simulink model "simulation_model"  (R2023a)
settings: Solver=FixedStepAuto  StartTime=0.0  StopTime=100  FixedStep=ts  RelTol=1e-3
undefined symbols (not defined in the file): a_1, a_2, eta_0, K_p, k_R, k_theta_d, k_theta_p, p, p_0, theta_d
libraries: simulink x2, simulink_extras x1
settings Model: Creator=mori_keigo  LastModifiedBy=mori_keigo

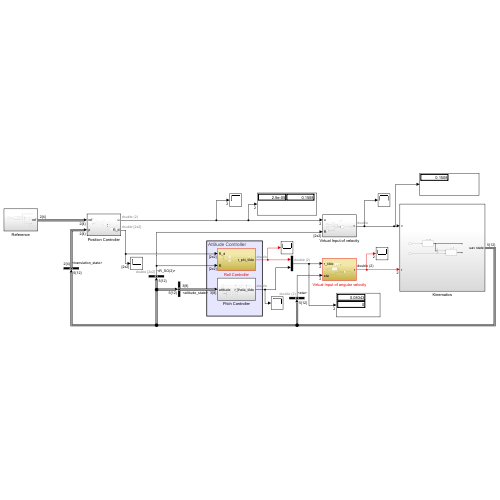
[thumbnail: Simulink's stored preview of the top-level diagram]
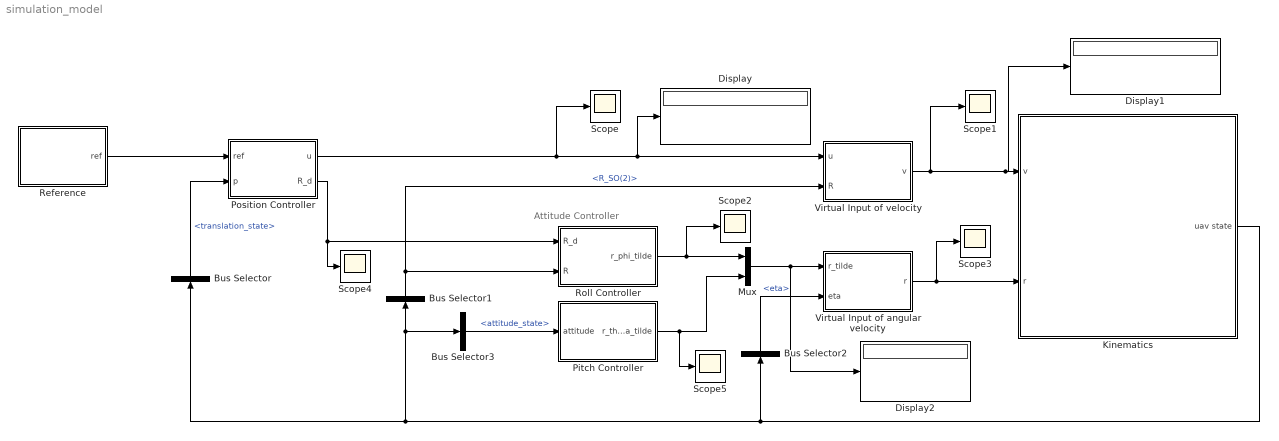
== system simulation_model ==
  note: Attitude Controller
  Bus Selector : BusSelector  OutputSignals=translation_state
  Bus Selector1 : BusSelector  OutputSignals=attitude_state.R_SO(2)
  Bus Selector2 : BusSelector  OutputSignals=attitude_state.eta
  Bus Selector3 : BusSelector  OutputSignals=attitude_state
  Display : Display
  Display1 : Display
  Display2 : Display
  Kinematics : Subsystem
  Mux : Mux  Inputs=2
  Pitch Controller : Subsystem
  Position Controller : Subsystem
  Reference : Subsystem
  Roll Controller : Subsystem
  Scope{,1..5} (6 alike) : Scope
  Virtual Input of angular velocity : Subsystem
  Virtual Input of velocity : Subsystem
  wires:
  Bus Selector/1 -> Position Controller/2(p)  "<translation_state>"
  Reference/1(ref) -> Position Controller/1(ref)
  Position Controller/1(u) -> Scope/1, Display/1, Virtual Input of velocity/1(u)
  Position Controller/2(R_d) -> Scope4/1, Roll Controller/1(R_d)
  Kinematics/1(uav state) -> Bus Selector/1, Bus Selector1/1, Bus Selector3/1, Bus Selector2/1
  Virtual Input of velocity/1(v) -> Display1/1, Kinematics/1(v), Scope1/1
  Roll Controller/1(r_phi_tilde) -> Scope2/1, Mux/1
  Pitch Controller/1(r_theta_tilde) -> Scope5/1, Mux/2
  Mux/1 -> Display2/1, Virtual Input of angular velocity/1(r_tilde)
  Virtual Input of angular velocity/1(r) -> Kinematics/2(r), Scope3/1
  Bus Selector3/1 -> Pitch Controller/1(attitude)  "<attitude_state>"
  Bus Selector1/1 -> Roll Controller/2(R), Virtual Input of velocity/2(R)  "<R_SO(2)>"
  Bus Selector2/1 -> Virtual Input of angular velocity/2(eta)  "<eta>"

== system simulation_model/Kinematics ==
  note: $\dot{\eta} = A \omega$
  note: $\dot{p} = Rv$
  v : Inport
  r : Inport  Port=2
  Bus Selector : BusSelector  OutputSignals=eta
  Kinematics of Attitude : Subsystem
  Kinematics of Translation : Subsystem
  Out Bus Element : Outport  PortName=uav state  Element=attitude_state
  Out Bus Element1 : Outport  PortName=uav state  Element=translation_state
  wires:
  r/1 -> Kinematics of Attitude/1(omega)
  v/1 -> Kinematics of Translation/2(v_z)
  Kinematics of Attitude/1(attitude_state) -> Bus Selector/1, Out Bus Element/1
  Kinematics of Translation/1(uav state) -> Out Bus Element1/1
  Bus Selector/1 -> Kinematics of Translation/1(eta)  "<eta>"

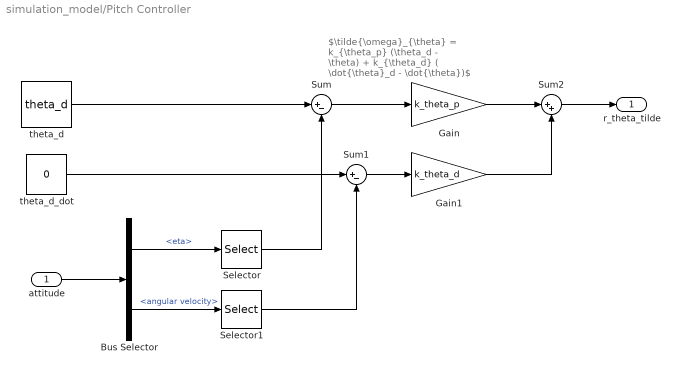
== system simulation_model/Pitch Controller ==
  note: $\tilde{\omega}_{\theta} = k_{\theta_p} (\theta_d - \theta) + k_{\theta_d} ( \dot{\theta}_d - \dot{\theta})$
  attitude : Inport
  Bus Selector : BusSelector  OutputSignals=eta,angular velocity
  Gain : Gain  Gain=k_theta_p
  Gain1 : Gain  Gain=k_theta_d
  Selector : Selector  InputPortWidth=2  IndexOptions=Index vector (dialog)  Indices=[2]  OutputSizes=1
  Selector1 : Selector  InputPortWidth=2  IndexOptions=Index vector (dialog)  Indices=[2]  OutputSizes=1
  Sum : Sum  Inputs=|+-
  Sum1 : Sum  Inputs=|+-
  Sum2 : Sum  Inputs=|++
  theta_d : Constant  Value=theta_d
  theta_d_dot : Constant  Value=0
  r_theta_tilde : Outport
  wires:
  attitude/1 -> Bus Selector/1
  theta_d/1 -> Sum/1
  theta_d_dot/1 -> Sum1/1
  Sum/1 -> Gain/1
  Sum1/1 -> Gain1/1
  Gain/1 -> Sum2/1
  Gain1/1 -> Sum2/2
  Sum2/1 -> r_theta_tilde/1
  Bus Selector/1 -> Selector/1  "<eta>"
  Selector/1 -> Sum/2
  Bus Selector/2 -> Selector1/1  "<angular velocity>"
  Selector1/1 -> Sum1/2

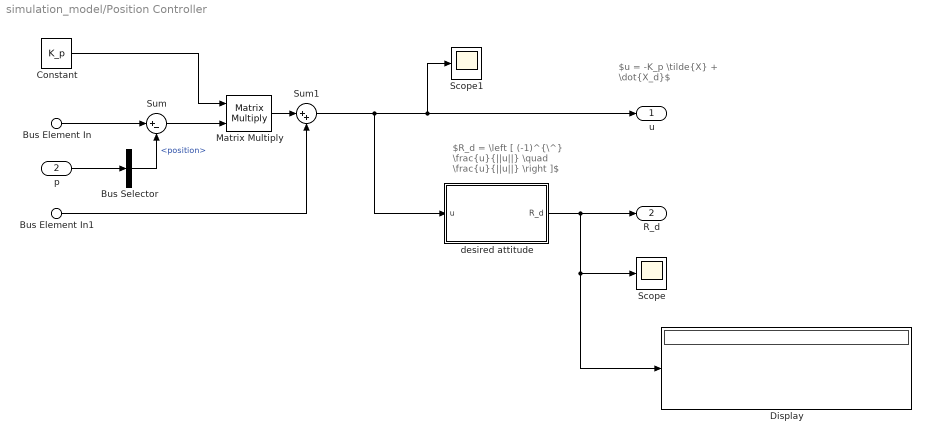
== system simulation_model/Position Controller ==
  note: $u = -K_p \tilde{X} + \dot{X_d}$
  note: $R_d = \left [ (-1)^{\^} \frac{u}{||u||} \quad \frac{u}{||u||} \right ]$
  Bus Element In : Inport  PortName=ref  Element=p_d
  Bus Element In1 : Inport  PortName=ref  Element=p_d_dot
  p : Inport  Port=2
  Bus Selector : BusSelector  OutputSignals=position
  Constant : Constant  Value=K_p
  Display : Display
  Matrix Multiply : Product  Multiplication=Matrix(*)
  Scope : Scope
  Scope1 : Scope
  Sum : Sum  Inputs=|+-
  Sum1 : Sum  Inputs=|++
  desired attitude : Subsystem
  u : Outport
  R_d : Outport  Port=2
  wires:
  Bus Element In/1 -> Sum/1
  Bus Element In1/1 -> Sum1/2
  desired attitude/1(R_d) -> R_d/1, Scope/1, Display/1
  Matrix Multiply/1 -> Sum1/1
  Constant/1 -> Matrix Multiply/1
  Sum/1 -> Matrix Multiply/2
  p/1 -> Bus Selector/1
  Bus Selector/1 -> Sum/2  "<position>"
  Sum1/1 -> u/1, Scope1/1, desired attitude/1(u)

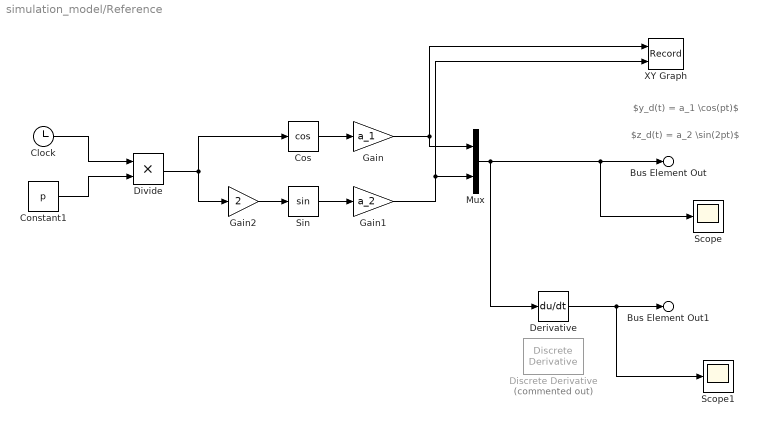
== system simulation_model/Reference ==
  note: $y_d(t) = a_1 \cos(pt)$
  note: $z_d(t) = a_2 \sin(2pt)$
  Clock : Clock
  Constant1 : Constant  Value=p
  Cos : Trigonometry  Operator=cos
  Derivative : Derivative
  Discrete Derivative : simulink/Discrete/Discrete Derivative  Commented=on  gainval=1.0  ICPrevScaledInput=0.0  OutMin=[]  OutMax=[]  OutDataType=fixdt(1, 16)  OutScaling=2^-10  DoSatur=off
  Divide : Product  Inputs=**
  Gain : Gain  Gain=a_1
  Gain1 : Gain  Gain=a_2
  Gain2 : Gain  Gain=2
  Mux : Mux  Inputs=2
  Scope : Scope
  Scope1 : Scope
  Sin : Trigonometry
  XY Graph : Record  FileSettingsInternal="{\"entries\":[{\"content\":{\"excelSettings\":{\"content\":{},\"type\":\"Streamout.ExcelSettings\"}},\"type\":\"Streamout.FileSettingStorage\",\"uuid\":\"\"}],\"packageUris\":[\"http:\\/\\/schema.mathworks.com\\/mf0\\/streamout_blocks\\/R2020a\"],\"version\":\"1.0\"}"  Layout=[1 1]  SignalsInternal="{\"entries\":[{\"content\":{\"signals\":[{\"content\":{\"blockPath\":[],\"dimensions\":[1],\"domain\":\"\",\"lineColor\":\"#a2142f\",\"plots\":[1],\"port\":1,\"sid\":[\"\"],\"signalID\":9636,\"signalName\":\"Gain\"},\"type\":\"RecordBlkView.Signal\",\"uuid\":\"\"},{\"content\":{\"blockPath\":[],\"dimensions\":[1],\"domain\":\"\",\"lineColor\":\"#139fff\",\"plots\":[1],\"port\":2,\"sid\":[\"\"],\"signalID\":9640,\"signalName\":\"Gain1\"},\"type\":\"RecordBlkView.Signal\",\"uuid\":\"\"}]},\"type\":\"RecordBlkView.InputSignals\",\"uuid\":\"\"}],\"packageUris\":[\"http:\\/\\/schema.mathworks.com\\/mf0\\/streamout_blocks\\/R2020a\"],\"version\":\"1.0\"}"  VisualizationBindings="{\"xyplotplugin\":{\"info\":[{\"series\":[{\"bindingParametersList\":[{\"parameter\":\"X-Axis\",\"signalID\":9636,\"signalName\":\"Gain\"},{\"parameter\":\"Y-Axis\",\"signalID\":9640,\"signalName\":\"Gain1\"}],\"seriesID\":31698}],\"subplotID\":1}]}}"  CompatibilityTag=XY
  Bus Element Out : Outport  PortName=ref  Element=p_d
  Bus Element Out1 : Outport  PortName=ref  Element=p_d_dot
  wires:
  Mux/1 -> Derivative/1, Scope/1, Bus Element Out/1
  Cos/1 -> Gain/1
  Sin/1 -> Gain1/1
  Constant1/1 -> Divide/2
  Clock/1 -> Divide/1
  Gain2/1 -> Sin/1
  Divide/1 -> Cos/1, Gain2/1
  Gain1/1 -> Mux/2, XY Graph/2
  Gain/1 -> XY Graph/1, Mux/1
  Derivative/1 -> Scope1/1, Bus Element Out1/1

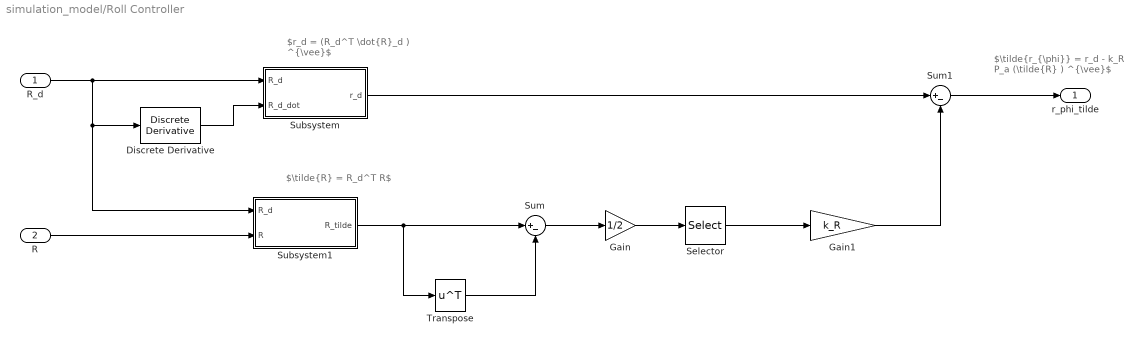
== system simulation_model/Roll Controller ==
  note: $r_d = (R_d^T \dot{R}_d ) ^{\vee}$
  note: $\tilde{r_{\phi}} = r_d - k_R P_a (\tilde{R} ) ^{\vee}$
  note: $\tilde{R} = R_d^T R$
  R_d : Inport
  R : Inport  Port=2
  Discrete Derivative : simulink/Discrete/Discrete Derivative  gainval=1.0  ICPrevScaledInput=0.0  OutMin=[]  OutMax=[]  OutDataType=fixdt(1, 16)  OutScaling=2^-10  DoSatur=off
  Gain : Gain  Gain=1/2
  Gain1 : Gain  Gain=k_R
  Selector : Selector  NumberOfDimensions=2  InputPortWidth=3  IndexOptions=Index vector (dialog),Index vector (dialog)  Indices=[2],1  OutputSizes=1,1
  Subsystem : Subsystem
  Subsystem1 : Subsystem
  Sum : Sum  Inputs=|+-
  Sum1 : Sum  Inputs=|+-
  Transpose : Math  Operator=transpose
  r_phi_tilde : Outport
  wires:
  R_d/1 -> Subsystem1/1(R_d), Discrete Derivative/1, Subsystem/1(R_d)
  Discrete Derivative/1 -> Subsystem/2(R_d_dot)
  R/1 -> Subsystem1/2(R)
  Subsystem1/1(R_tilde) -> Transpose/1, Sum/1
  Transpose/1 -> Sum/2
  Sum/1 -> Gain/1
  Gain/1 -> Selector/1
  Selector/1 -> Gain1/1
  Sum1/1 -> r_phi_tilde/1
  Subsystem/1(r_d) -> Sum1/1
  Gain1/1 -> Sum1/2

== system simulation_model/Virtual Input of angular velocity ==
  note: $r = A^{-1} \tilde{r}$
  r_tilde : Inport
  eta : Inport  Port=2
  Product : Product  Inputs=/*  Multiplication=Matrix(*)
  Transformation to A : Subsystem
  r : Outport
  wires:
  Transformation to A/1(A) -> Product/1
  r_tilde/1 -> Product/2
  Product/1 -> r/1
  eta/1 -> Transformation to A/1(eta)

== system simulation_model/Virtual Input of velocity ==
  note: $v_z = u^T Re_2$
  u : Inport
  R : Inport  Port=2
  Constant : Constant  Value=[0;1]  VectorParams1D=off
  Matrix Multiply : Product  Inputs=3  Multiplication=Matrix(*)
  Transpose : Math  Operator=transpose
  v : Outport
  wires:
  R/1 -> Matrix Multiply/2
  Transpose/1 -> Matrix Multiply/1
  Matrix Multiply/1 -> v/1
  u/1 -> Transpose/1
  Constant/1 -> Matrix Multiply/3

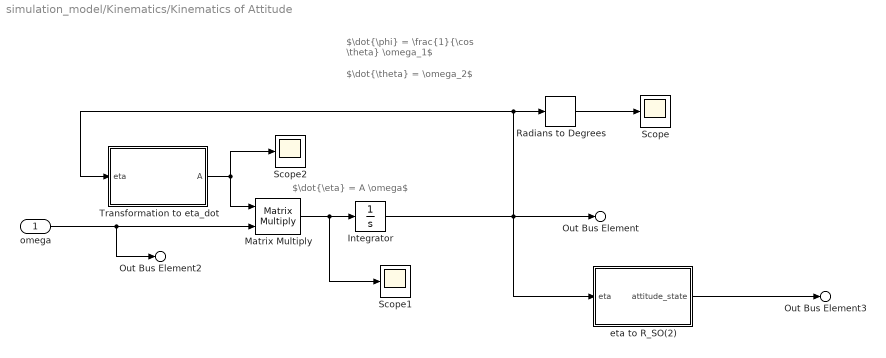
== system simulation_model/Kinematics/Kinematics of Attitude ==
  note: $\dot{\theta} = \omega_2$
  note: $\dot{\phi} = \frac{1}{\cos \theta} \omega_1$
  note: $\dot{\eta} = A \omega$
  omega : Inport
  Integrator : Integrator  InitialCondition=eta_0
  Matrix Multiply : Product  Multiplication=Matrix(*)
  Radians to Degrees : simulink_extras/Transformations/Radians to Degrees
  Scope : Scope
  Scope1 : Scope
  Scope2 : Scope
  Transformation to eta_dot : Subsystem
  eta to R_SO(2) : Subsystem
  Out Bus Element : Outport  PortName=attitude_state  Element=eta
  Out Bus Element2 : Outport  PortName=attitude_state  Element=angular velocity
  Out Bus Element3 : Outport  PortName=attitude_state  Element=R_SO(2)
  wires:
  Integrator/1 -> Out Bus Element/1, eta to R_SO(2)/1(eta), Transformation to eta_dot/1(eta), Radians to Degrees/1
  Matrix Multiply/1 -> Scope1/1, Integrator/1
  omega/1 -> Out Bus Element2/1, Matrix Multiply/2
  Transformation to eta_dot/1(A) -> Matrix Multiply/1, Scope2/1
  Radians to Degrees/1 -> Scope/1
  eta to R_SO(2)/1(attitude_state) -> Out Bus Element3/1

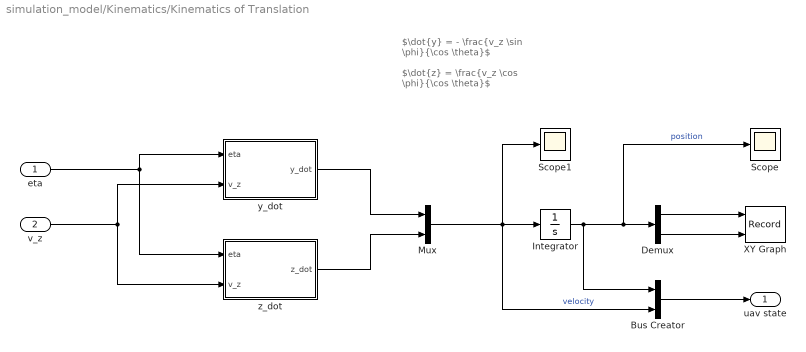
== system simulation_model/Kinematics/Kinematics of Translation ==
  note: $\dot{z} = \frac{v_z \cos \phi}{\cos \theta}$
  note: $\dot{y} = - \frac{v_z \sin \phi}{\cos \theta}$
  eta : Inport
  v_z : Inport  Port=2
  Bus Creator : BusCreator  Inputs=2
  Demux : Demux  Outputs=2
  Integrator : Integrator  InitialCondition=p_0
  Mux : Mux  Inputs=2
  Scope : Scope
  Scope1 : Scope
  XY Graph : Record  FileSettingsInternal="{\"entries\":[{\"content\":{\"excelSettings\":{\"content\":{},\"type\":\"Streamout.ExcelSettings\"}},\"type\":\"Streamout.FileSettingStorage\",\"uuid\":\"\"}],\"packageUris\":[\"http:\\/\\/schema.mathworks.com\\/mf0\\/streamout_blocks\\/R2020a\"],\"version\":\"1.0\"}"  Layout=[1 1]  SignalsInternal="{\"entries\":[{\"content\":{\"signals\":[{\"content\":{\"blockPath\":[],\"dimensions\":[1],\"domain\":\"\",\"lineColor\":\"#a2142f\",\"plots\":[1],\"port\":1,\"sid\":[\"\"],\"signalID\":9628,\"signalName\":\"Demux:1\"},\"type\":\"RecordBlkView.Signal\",\"uuid\":\"\"},{\"content\":{\"blockPath\":[],\"dimensions\":[1],\"domain\":\"\",\"lineColor\":\"#139fff\",\"plots\":[1],\"port\":2,\"sid\":[\"\"],\"signalID\":9632,\"signalName\":\"Demux:2\"},\"type\":\"RecordBlkView.Signal\",\"uuid\":\"\"}]},\"type\":\"RecordBlkView.InputSignals\",\"uuid\":\"\"}],\"packageUris\":[\"http:\\/\\/schema.mathworks.com\\/mf0\\/streamout_blocks\\/R2020a\"],\"version\":\"1.0\"}"  VisualizationBindings="{\"xyplotplugin\":{\"info\":[{\"series\":[{\"bindingParametersList\":[{\"parameter\":\"X-Axis\",\"signalID\":9628,\"signalName\":\"Demux:1\"},{\"parameter\":\"Y-Axis\",\"signalID\":9632,\"signalName\":\"Demux:2\"}],\"seriesID\":17287}],\"subplotID\":1}]}}"  CompatibilityTag=XY
  y_dot : Subsystem
  z_dot : Subsystem
  uav state : Outport
  wires:
  Integrator/1 -> Scope/1, Demux/1, Bus Creator/1  "position"
  Mux/1 -> Scope1/1, Bus Creator/2, Integrator/1  "velocity"
  Bus Creator/1 -> uav state/1
  eta/1 -> z_dot/1(eta), y_dot/1(eta)
  y_dot/1(y_dot) -> Mux/1
  v_z/1 -> z_dot/2(v_z), y_dot/2(v_z)
  z_dot/1(z_dot) -> Mux/2
  Demux/1 -> XY Graph/1
  Demux/2 -> XY Graph/2

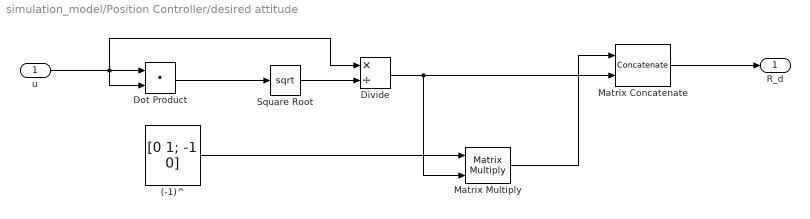
== system simulation_model/Position Controller/desired attitude ==
  u : Inport
  (-1)^ : Constant  Value=[0 1; -1 0]  VectorParams1D=off
  Divide : Product  Inputs=*/
  Dot Product : DotProduct  OutDataTypeStr=Inherit: Inherit via internal rule
  Matrix Concatenate : Concatenate  Mode=Multidimensional array  ConcatenateDimension=2
  Matrix Multiply : Product  Multiplication=Matrix(*)
  Square Root : Sqrt
  R_d : Outport
  wires:
  Dot Product/1 -> Square Root/1
  u/1 -> Divide/1, Dot Product/2, Dot Product/1
  Square Root/1 -> Divide/2
  Matrix Concatenate/1 -> R_d/1
  Divide/1 -> Matrix Concatenate/2, Matrix Multiply/2
  (-1)^/1 -> Matrix Multiply/1
  Matrix Multiply/1 -> Matrix Concatenate/1

== system simulation_model/Roll Controller/Subsystem ==
  R_d : Inport
  R_d_dot : Inport  Port=2
  Matrix Multiply : Product  Multiplication=Matrix(*)
  Selector : Selector  NumberOfDimensions=2  InputPortWidth=3  IndexOptions=Index vector (dialog),Index vector (dialog)  Indices=[2],1  OutputSizes=1,1
  Transpose : Math  Operator=transpose
  r_d : Outport
  wires:
  R_d/1 -> Transpose/1
  Transpose/1 -> Matrix Multiply/1
  R_d_dot/1 -> Matrix Multiply/2
  Matrix Multiply/1 -> Selector/1
  Selector/1 -> r_d/1

== system simulation_model/Roll Controller/Subsystem1 ==
  R_d : Inport
  R : Inport  Port=2
  Matrix Multiply : Product  Multiplication=Matrix(*)
  Transpose : Math  Operator=transpose
  R_tilde : Outport
  wires:
  R_d/1 -> Transpose/1
  Transpose/1 -> Matrix Multiply/1
  R/1 -> Matrix Multiply/2
  Matrix Multiply/1 -> R_tilde/1

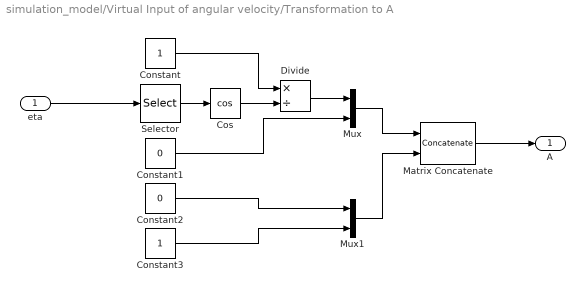
== system simulation_model/Virtual Input of angular velocity/Transformation to A ==
  eta : Inport
  Constant : Constant
  Constant1 : Constant  Value=0
  Constant2 : Constant  Value=0
  Constant3 : Constant
  Cos : Trigonometry  Operator=cos
  Divide : Product  Inputs=*/
  Matrix Concatenate : Concatenate  Mode=Multidimensional array  ConcatenateDimension=2
  Mux : Mux  Inputs=2
  Mux1 : Mux  Inputs=2
  Selector : Selector  InputPortWidth=2  IndexOptions=Index vector (dialog)  Indices=[2]  OutputSizes=1
  A : Outport
  wires:
  eta/1 -> Selector/1
  Constant/1 -> Divide/1
  Divide/1 -> Mux/1
  Constant1/1 -> Mux/2
  Constant2/1 -> Mux1/1
  Constant3/1 -> Mux1/2
  Mux/1 -> Matrix Concatenate/1
  Mux1/1 -> Matrix Concatenate/2
  Matrix Concatenate/1 -> A/1
  Selector/1 -> Cos/1
  Cos/1 -> Divide/2

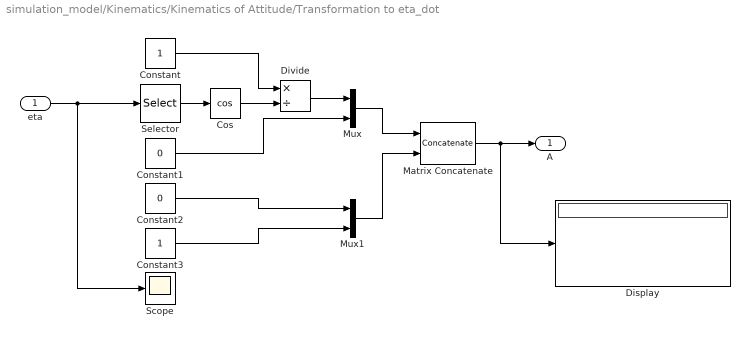
== system simulation_model/Kinematics/Kinematics of Attitude/Transformation to eta_dot ==
  eta : Inport
  Constant : Constant
  Constant1 : Constant  Value=0
  Constant2 : Constant  Value=0
  Constant3 : Constant
  Cos : Trigonometry  Operator=cos
  Display : Display
  Divide : Product  Inputs=*/
  Matrix Concatenate : Concatenate  Mode=Multidimensional array  ConcatenateDimension=2
  Mux : Mux  Inputs=2
  Mux1 : Mux  Inputs=2
  Scope : Scope
  Selector : Selector  InputPortWidth=2  IndexOptions=Index vector (dialog)  Indices=[2]  OutputSizes=1
  A : Outport
  wires:
  eta/1 -> Scope/1, Selector/1
  Constant/1 -> Divide/1
  Divide/1 -> Mux/1
  Constant1/1 -> Mux/2
  Constant2/1 -> Mux1/1
  Constant3/1 -> Mux1/2
  Mux/1 -> Matrix Concatenate/1
  Mux1/1 -> Matrix Concatenate/2
  Matrix Concatenate/1 -> Display/1, A/1
  Selector/1 -> Cos/1
  Cos/1 -> Divide/2

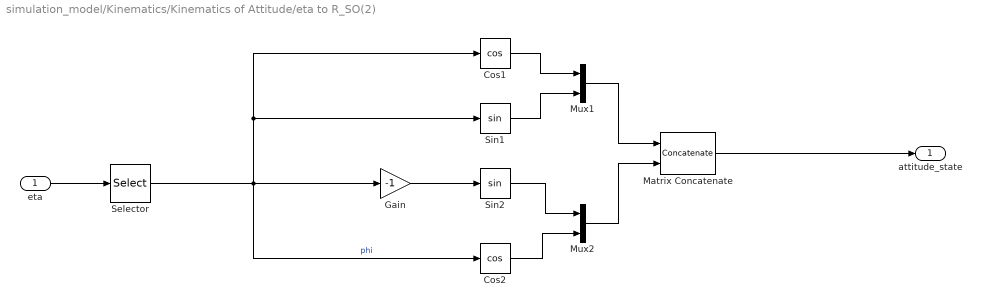
== system simulation_model/Kinematics/Kinematics of Attitude/eta to R_SO(2) ==
  eta : Inport
  Cos1 : Trigonometry  Operator=cos
  Cos2 : Trigonometry  Operator=cos
  Gain : Gain  Gain=-1
  Matrix Concatenate : Concatenate  Mode=Multidimensional array  ConcatenateDimension=2
  Mux1 : Mux  Inputs=2
  Mux2 : Mux  Inputs=2
  Selector : Selector  InputPortWidth=2  IndexOptions=Index vector (dialog)  Indices=[1]  OutputSizes=1
  Sin1 : Trigonometry
  Sin2 : Trigonometry
  attitude_state : Outport
  wires:
  eta/1 -> Selector/1
  Cos2/1 -> Mux2/2
  Matrix Concatenate/1 -> attitude_state/1
  Mux2/1 -> Matrix Concatenate/2
  Mux1/1 -> Matrix Concatenate/1
  Gain/1 -> Sin2/1
  Cos1/1 -> Mux1/1
  Sin2/1 -> Mux2/1
  Sin1/1 -> Mux1/2
  Selector/1 -> Cos2/1, Gain/1, Cos1/1, Sin1/1  "phi"

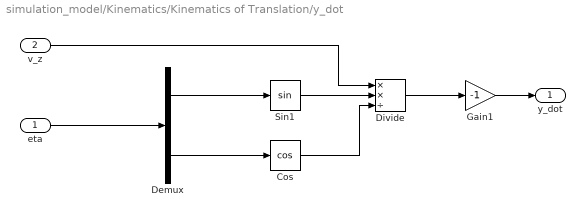
== system simulation_model/Kinematics/Kinematics of Translation/y_dot ==
  eta : Inport
  v_z : Inport  Port=2
  Cos : Trigonometry  Operator=cos
  Demux : Demux  Outputs=2
  Divide : Product  Inputs=**/
  Gain1 : Gain  Gain=-1
  Sin1 : Trigonometry
  y_dot : Outport
  wires:
  Demux/1 -> Sin1/1
  Sin1/1 -> Divide/2
  v_z/1 -> Divide/1
  Demux/2 -> Cos/1
  Cos/1 -> Divide/3
  eta/1 -> Demux/1
  Gain1/1 -> y_dot/1
  Divide/1 -> Gain1/1

== system simulation_model/Kinematics/Kinematics of Translation/z_dot ==
  eta : Inport
  v_z : Inport  Port=2
  Cos1 : Trigonometry  Operator=cos
  Cos2 : Trigonometry  Operator=cos
  Demux : Demux  Outputs=2
  Divide : Product  Inputs=**/
  z_dot : Outport
  wires:
  eta/1 -> Demux/1
  Demux/1 -> Cos2/1
  Demux/2 -> Cos1/1
  v_z/1 -> Divide/1
  Cos2/1 -> Divide/2
  Cos1/1 -> Divide/3
  Divide/1 -> z_dot/1
